simulink model "Buck_Boost_Converter_Model"  (R2020a)
settings: Solver=VariableStepAuto  StartTime=0.0  StopTime=1  RelTol=1e-3
libraries: powerlib x8, powerlib_meascontrol x1
settings Model: Creator=Ricardo Romero  LastModifiedBy=Ricardo Romero

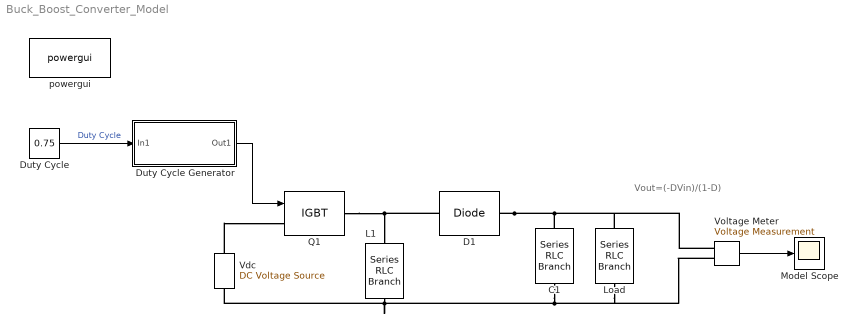
== system Buck_Boost_Converter_Model ==
  note: Vout=(-DVin)/(1-D)
  C1 : powerlib/Elements/Series RLC Branch  LConnTagsString=__new0  RConnTagsString=__new0  BranchType=C  Resistance=1  Inductance=1e-3  SetiL0=off  InitialCurrent=0  Capacitance=10e-3  Setx0=off  InitialVoltage=0  Measurements=None
  D1 : powerlib/Power Electronics/Diode  Ron=0.001  Lon=0  Vf=0.8  IC=0  UseSnubber=0  Rs=500  Cs=250e-9  Measurements=off
  Duty Cycle : Constant  Value=0.75
  Duty Cycle Generator : Subsystem
  L1 : powerlib/Elements/Series RLC Branch  LConnTagsString=__new0  RConnTagsString=__new0  BranchType=L  Resistance=1  Inductance=1e-3  SetiL0=off  InitialCurrent=0  Capacitance=1e-6  Setx0=off  InitialVoltage=0  Measurements=None
  Load : powerlib/Elements/Series RLC Branch  LConnTagsString=__new0  RConnTagsString=__new0  BranchType=R  Resistance=10  Inductance=1e-3  SetiL0=off  InitialCurrent=0  Capacitance=1e-6  Setx0=off  InitialVoltage=0  Measurements=None
  Model Scope : Scope
  Q1 : powerlib/Power Electronics/IGBT  Ron=0.001  Lon=0  Vf=1  Tf=1e-6  Tt=2e-6  IC=0  Rs=1e5  Cs=inf  Measurements=off
  Vdc : powerlib/Electrical Sources/DC Voltage Source  Amplitude=10  Measurements=None
  Voltage Meter : powerlib/Measurements/Voltage Measurement  PhasorSimulation=off  OutputType=Complex  PSBequivalent=0
  powergui : powerlib/powergui  Priority=1  SimulationMode=Continuous  SampleTime=50e-6  frequency=60  Iterations=50  frequencyindice=0  Pbase=100e6  ErrMax=1e-4  UnitsV=kV  UnitsW=MW  buscounter=0  FunctionMessages=off  echomessages=off  EnableUseOfTLC=off  CurrentSourceSwitches=off  DisableSnubberDevices=off  DisableRonSwitches=off  DisableVfSwitches=off  DisplayEquations=off  AutomaticDiscreteSolvers=off  SolverType=Tustin/Backward Euler (TBE)  Interpol=off  ExternalGateDelay=off  methode=off  Ts=100  x0status=blocks  SPID=on  SwTol=0  HookPort=off  NonlinearTolerance=1e-4  nMaxIteration=100  ContinueOnMaxIteration=off  RestoreLinks=warning  ResistiveCurrentMeasurement=off  Frange=[0:2:500]  Ylog=off  Xlog=on  ShowGrid=off  save=off  variable=ZData  structure=0  ZoomFFT=off  StartTime=0.0  cycles=1  DisplayStyle=1  fundamental=60  FreqAxis=off  MaxFrequency=1000  frequencyindicesteady=1  RmsSteady=1  display=off
  wires:
  Duty Cycle/1 -> Duty Cycle Generator/1(In1)  "Duty Cycle"
  Voltage Meter/1 -> Model Scope/1
  Duty Cycle Generator/1(Out1) -> Q1/1
  connections:
  Vdc/RConn1 -- Q1/LConn1
  Q1/RConn1 -- L1/LConn1 -- D1/RConn1
  L1/RConn1 -- Voltage Meter/LConn1 -- Load/LConn1 -- C1/LConn1 -- Vdc/LConn1
  D1/LConn1 -- Voltage Meter/LConn2 -- Load/RConn1 -- C1/RConn1

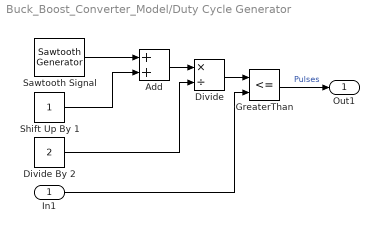
== system Buck_Boost_Converter_Model/Duty Cycle Generator ==
  In1 : Inport
  Add : Sum
  Divide : Product  Inputs=*/
  Divide By 2 : Constant  Value=2
  GreaterThan : RelationalOperator  Operator=<=  OutDataTypeStr=boolean  RndMeth=Simplest
  Sawtooth Signal : powerlib_meascontrol/Pulse & Signal Generators/Sawtooth Generator  Freq=5e3  Phase=0  Ts=0
  Shift Up By 1 : Constant
  Out1 : Outport
  wires:
  Divide/1 -> GreaterThan/1
  GreaterThan/1 -> Out1/1  "Pulses"
  Divide By 2/1 -> Divide/2
  Sawtooth Signal/1 -> Add/1
  Add/1 -> Divide/1
  Shift Up By 1/1 -> Add/2
  In1/1 -> GreaterThan/2
